simulink library "slident"  (Simulink 7.5)
settings: Solver=ode45  SolverMode=SingleTasking  StartTime=0.0  StopTime=10.0  RelTol=1e-3
values from neighbouring files (symbols this model uses):
  A = (pinv(R2(1:n,1:n)) * R2(1:n,n+1)).'    [ar.m]    (also in motor.m = s(1:2,1:2); n4sid.m = stab(A))
  B = s(1:2,3)    [motor.m]    (also in n4sid.m = B1)
  C = eye(2)    [motor.m]    (also in n4sid.m = conj(Un(1:ny,1:n)))
  D = D .* abs(ec{kexp}*ones(1,size(D,2)))    [arx.m]    (also in ivx.m = (OM(inda,:).').*(-Y*ones(1,na)); motor.m = [0;0]; n4sid.m = D1)
  data = pvset(data,'Name',Name)    [ar.m]    (also in arx.m = complex(data); arx_f.m = data(:,:,[]); etfe.m = iddata(data,[],T); idfilt.m = zfc{1})
  ts = ts{1}    [arx.m]    (also in arx_f.m = ts{1};[num1,den1]=tfdata(m0); arxstruc.m = pvget(z,'Ts'); iv4.m; n4sid.m)
  Ts = pvget(m0,'Ts')    [arx.m]    (also in arx_f.m = Ts{1}; idfilt.m = {1}; idresamp.m = pvget(data,'Ts'); iv4.m = Ts{1})
  X0 = [0;0]    [motor.m]    (also in n4sid.m = x(nxr,:).')
undefined symbols (not defined in the file or in its folder): Demos, gcbh, iddata, idss, idutils, offset, ph, slident2, Tdi, tsn
libraries: simulink x1
settings Model: RequirementInfo=9  Creator=greg  LastModifiedBy=rsingh  ExtModeAutoUpdateStatusClock=off
settings Model: ForwardingTableString=|
  | ||__slOldName__||slident/Output-error
  | model estimator.||__slNewName__||slident/Output-error
  | model estimator||__slOldName__||slident/Idnlgrey Model||__slNewName__||slident/Nonlinear Grey-Box Model

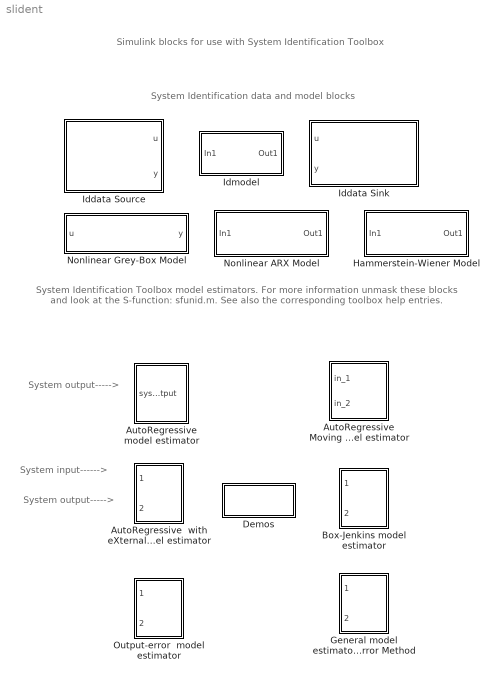
== system slident ==
  note: System Identification data and model blocks
  note: System output----->
  note: System input------>
  note: System output----->
  note: System Identification Toolbox model estimators. For more information
      | unmask these blocks and look at the  S-function: sfunid.m.
      | See also the corresponding toolbox help entries.
  note: Simulink blocks for use with
      | System Identification Toolbox
  AutoRegressive model estimator : Subsystem  AncestorBlock=slident2/AutoRegressive model estimator  mask(AR){order=3, HowOften=25, tso=0.05, npts=200, mn=, cbsim=1 step prediction}
      mask prompts: order "Orders of model [na]:"; HowOften "How often to update model (samples):"; tso "Sample time:"; npts "Length of data window (samples):"; mn "Model name:"; cbsim "Prediction horizon:"
      mask help:
      | Autoregressive model estimator for a scalar valued signal.
      | Model Name: Enter workspace variable name for resulting models. Leave empty for printout to MATLAB Command Window.
      | Choose prediction-horizon for the plots.
      mask init:
      | method='ar';
      | [ts,offset,ph,mn]=slidentinit(tso,cbsim,mn);
      mask Help:
      | AR block facilitates estimation of auto-regressive models in Simulink(R). Type "help ar" for more information. <br>
      | 
      | <p>
      | Hook a data source block to the input of the AR block. The estimated models are based on the latest data in the Data window. (initially padded with zeros). The model is re-estimated at the chosen rate. </p>
      | <p>
      | If a Model Name M is entered, the variable M will contain the estimated models
      | in a cell array, so that M{k,1} is the time associated with the k:th model and
      | M{k,2} is the actual model in IDPOLY format. The models can be used in Simulink(R) for simulation using the Idmodel block. They can also be simulated, analyzed and transformed in MATLAB Command Window using commands available with System Identification Toolbox(TM). For example, bode(M{:;2}) and step(M{:,2}) will show the bode plots and step responses of all the models.
      | </p>
      | <p>
      | If the model name is left empty, the models will be displayed in MATLAB Command Window. The properties of the models will also be displayed, on-line, as the  predicted output of the current model compared with the measured (actual) data. Choose between various prediction horizons using the Prediction horizon popup menu of the AR block. </p>
      | 
      | <p>
      | Results are displayed as the one step ahead predicted output versus the true output in graphical form.</p>
      mask StyleString: edit,edit,edit,edit,edit,popup(1 step prediction|5 step prediction|10 step prediction)
      mask Display:
      | disp('AR')
      | port_label('input',1,'y')
  AutoRegressive  with eXternal input model estimator : Subsystem  AncestorBlock=|  mask(ARX){order=[2 2 1], HowOften=25, tso=0.05, npts=200, mn=, cbsim=Simulation}
      | slident2/AutoRegressive 
      | with eXternal input
      | model estimator
      mask prompts: order "Orders of model [na nb nk]:"; HowOften "How often update model (samples):"; tso "Sample time:"; npts "Length of data window (samples):"; mn "Model name:"; cbsim "Simulation/Prediction:"
      mask help:
      | ARX model estimator.
      | Hook input 1 to system input.
      | Hook input 2 to system output.
      | Model Name: Enter workspace variable name for resulting models. Leave empty for printout to MATLAB Command Window.
      | Choose if presented model plots should be for simulation or prediction.
      mask init:
      | method='arx';
      | [ts,offset,ph,mn]=slidentinit(tso,cbsim,mn);
      mask Help:
      | ARX block facilitates estimation of auto-regressive models with exogenous inputs in Simulink(R). Type "help arx" for more information. <br>
      | 
      | <p>
      | Hook a data source representing input to an actual system to the first port of this block. Hook a data source representing measured output of the system to second port of the block. The estimated models are based on the latest data in the Data window. (initially padded with zeros). The model is re-estimated at the chosen rate. </p>
      | 
      | <p>
      | If a Model Name M is entered, the variable M will contain the estimated models
      | in a cell array, so that M{k,1} is the time associated with the k:th model and
      | M{k,2} is the actual model in IDPOLY format. The models can be used in Simulink(R) for simulation using the Idmodel block. They can also be simulated, analyzed and transformed in MATLAB Command Window using commands available with System Identification Toolbox(TM). For example, bode(M{:;2}) and step(M{:,2}) will show the bode plots and step responses of all the models. </p>
      | 
      | <p>
      | If the model name is left empty, the models will be displayed in MATLAB Command Window.
      | The properties of the models will also be displayed, on-line, as the simulated/predicted
      | output of the current model, compared with the measured (actual) output. Choose between
      | simulated outputs and predicted outputs over various prediction horizons. </p>
      mask StyleString: edit,edit,edit,edit,edit,popup(Simulation|1 step prediction|5 step prediction|10 step prediction)
      mask Display:
      | disp('ARX')
      | port_label('input',1,'u')
      | port_label('input',2,'y')
  AutoRegressive Moving Average with eXternal input model estimator : Subsystem  AncestorBlock=|  mask(ARMAX){order=[2 2 2 1], HowOften=25, tso=0.05, npts=200, mn=, cbsim=Simulation}
      | slident2/AutoRegressive Moving
      | Average with eXternal
      | input model estimator
      mask prompts: order "Orders of model [na nb nc nk]:"; HowOften "How often to update model (samples):"; tso "Sample time:"; npts "Length of data window (samples):"; mn "Model name:"; cbsim "Simulation/Prediction:"
      mask help:
      | ARMAX model estimator.
      | Hook input 1 to system input.
      | Hook input 2 to system output.
      | Model Name: Enter workspace variable name for resulting models. Leave empty for printout to MATLAB Command Window.
      | Choose if presented model plots should be for simulation or prediction.
      mask init:
      | method='armax';
      | [ts,offset,ph,mn]=slidentinit(tso,cbsim,mn);
      mask Help:
      | ARMAX block facilitates estimation of auto-regressive, moving average models with inputs (ARMAX) in Simulink(R). Type "help armax" for more information. <br>
      | 
      | <p>
      | Hook a data source representing input to an actual system to the first port of this block. Hook a data source representing measured output of the system to second port of the block. The estimated models are based on the latest data in the Data window. (initially padded with zeros). The model is re-estimated at the chosen rate. </p>
      | 
      | <p>
      | If a Model Name M is entered, the variable M will contain the estimated models
      | in a cell array, so that M{k,1} is the time associated with the k:th model and
      | M{k,2} is the actual model in IDPOLY format. The models can be used in Simulink(R) for simulation using the Idmodel block. They can also be simulated, analyzed and transformed in MATLAB Command Window using commands available with System Identification Toolbox(TM). For example, bode(M{:;2}) and step(M{:,2}) will show the bode plots and step responses of all the models. </p>
      | 
      | <p>
      | If the model name is left empty, the models will be displayed in MATLAB Command Window.
      | The properties of the models will also be displayed, on-line, as the simulated/predicted
      | output of the current model, compared with the measured (actual) output. Choose between
      | simulated outputs and predicted outputs over various prediction horizons. </p>
      mask StyleString: edit,edit,edit,edit,edit,popup(Simulation|1 step prediction|5 step prediction|10 step prediction)
      mask Display:
      | disp('ARMAX')
      | port_label('input',1,'u')
      | port_label('input',2,'y')
  Box-Jenkins model estimator : Subsystem  AncestorBlock=slident2/Box-Jenkins model estimator  mask(BJ){order=[2 2 2 2 1], HowOften=25, tso=0.05, npts=200, mn=, cbsim=Simulation}
      mask prompts: order "Orders of model [nb nc nd nf nk]:"; HowOften "How often to update model (samples):"; tso "Sample time:"; npts "Length of data window:"; mn "Model name:"; cbsim "Simulation/Prediction:"
      mask help:
      | Box-Jenkins model estimator.
      | Hook input 1 to system input.
      | Hook input 2 to system output.
      | Model Name: Enter workspace variable name for resulting models. Leave empty for printout to MATLAB Command Window.
      | Choose if presented model plots should be for simulation or prediction.
      mask init:
      | method='bj';
      | [ts,offset,ph,mn]=slidentinit(tso,cbsim,mn);
      mask Help:
      | BJ block facilitates estimation of Box-Jenkins models in Simulink(R). Type "help bj" for more information. <br>
      | 
      | <p>
      | Hook a data source representing input to an actual system to the first port of this block. Hook a data source representing measured output of the system to second port of the block. The estimated models are based on the latest data in the Data window. (initially padded with zeros). The model is re-estimated at the chosen rate. </p>
      | 
      | <p>
      | If a Model Name M is entered, the variable M will contain the estimated models
      | in a cell array, so that M{k,1} is the time associated with the k:th model and
      | M{k,2} is the actual model in IDPOLY format. The models can be used in Simulink(R) for simulation using the Idmodel block. They can also be simulated, analyzed and transformed in MATLAB Command Window using commands available with System Identification Toolbox(TM). For example, bode(M{:;2}) and step(M{:,2}) will show the bode plots and step responses of all the models. </p>
      | 
      | <p>
      | If the model name is left empty, the models will be displayed in MATLAB Command Window.
      | The properties of the models will also be displayed, on-line, as the simulated/predicted
      | output of the current model, compared with the measured (actual) output. Choose between
      | simulated outputs and predicted outputs over various prediction horizons. </p>
      mask StyleString: edit,edit,edit,edit,edit,popup(Simulation|1 step prediction|5 step prediction|10 step prediction)
      mask Display:
      | disp('BJ')
      | port_label('input',1,'u')
      | port_label('input',2,'y')
  Demos : Subsystem  AncestorBlock=slident2/Demos
      settings: OpenFcn=demo('toolbox','system identification')
      mask Display: disp('Demos')
  General model estimator using Predictive Error Method : Subsystem  AncestorBlock=|  mask(PEM){order=[2 2 2 2 2 1], HowOften=25, tso=0.05, npts=200, mn=, cbsim=Simulation}
      | slident2/General model
      | estimator using
      | Predictive Error Method
      mask prompts: order "Orders of model [na nb nc nd nf nk]:"; HowOften "How often to update model (samples):"; tso "Sample time:"; npts "Length of data window (samples):"; mn "Model name:"; cbsim "Simulation/Prediction:"
      mask help:
      | General SISO polynomial model estimator.
      | Hook input 1 to system input.
      | Hook input 2 to system output.
      | Model Name: Enter workspace variable name for resulting models. Leave empty for printout to MATLAB Command Window.
      | Choose if presented model plots should be for simulation or prediction.
      mask init:
      | method='pem';
      | [ts,offset,ph,mn]=slidentinit(tso,cbsim,mn);
      mask Help:
      | PEM block facilitates estimation of generic linear polynomial models in Simulink(R). Only linear, SISO models are supported. A generic polynomial structure has all its coefficients active so that the model equation is: A y(t) = B/F u(t-Nk) + C/D e(t). Type "help pem" and "help idpoly" for more information. <br>
      | <p>
      | Hook a data source representing input to an actual system to the first port of this block. Hook a data source representing measured output of the system to second port of the block. The estimated models are based on the latest data in the Data window. (initially padded with zeros). The model is re-estimated at the chosen rate. </p>
      | 
      | <p>
      | If a Model Name M is entered, the variable M will contain the estimated models
      | in a cell array, so that M{k,1} is the time associated with the k:th model and
      | M{k,2} is the actual model in IDPOLY format. The models can be used in Simulink(R) for simulation using the Idmodel block. They can also be simulated, analyzed and transformed in MATLAB Command Window using commands available with System Identification Toolbox(TM). For example, bode(M{:;2}) and step(M{:,2}) will show the bode plots and step responses of all the models. </p>
      | 
      | <p>
      | If the model name is left empty, the models will be displayed in MATLAB Command Window.
      | The properties of the models will also be displayed, on-line, as the simulated/predicted
      | output of the current model, compared with the measured (actual) output. Choose between
      | simulated outputs and predicted outputs over various prediction horizons. </p>
      mask StyleString: edit,edit,edit,edit,edit,popup(Simulation|1 step prediction|5 step prediction|10 step prediction)
      mask Display:
      | disp('PEM')
      | port_label('input',1,'u')
      | port_label('input',2,'y')
  Hammerstein-Wiener Model : Subsystem  mask(Hammerstein-Wiener Model){sys=, IC=Zero, X0i=0}
      mask prompts: sys "Model"; IC "Initial conditions:"; X0i "Specify a vector of state values"
      mask help:
      | Simulate a Hammerstein-Wiener (idnlhw) model. Enter a valid variable or expression representing an idnlhw model for the field "Model". The initial conditions for simulation can be specified using one of the following ways:
      | 1. Use "Zero" to use a value of zero for all initial state values.
      | 2. Specify the initial state values explicitly as a numerical vector for the linear block of the idnlhw model. Click on Help button for information on computation of initial states.
      mask init:
      | MaskVal = get_param(gcb,'MaskValues');
      | sysname = MaskVal{1};
      | if isa(sys,'idnlhw')
      |     %sysname = MaskVal{1};
      | else
      |     if isempty(sysname)
      |         sysname = 'IDNLHW MODEL';
      |     else
      |         sysname = '???';
      |     end
      |     sys = [];
      |     X0i = [];
      | end
      | if any(strcmp(get_param(bdroot(gcb),'SimulationStatus'),{'initializing','updating'}))
      |     lwarn = lastwarn;warn = warning('off');
      |     try
      |         [A,B,C,D,X0,Ts,WarnMsg] = idnlhwmaskinit('initialization',gcb,sys,IC,X0i);
      |         warning(warn);lastwarn(lwarn);
      |         warning(WarnMsg)
      |     catch E
      |         sys = [];
      |         X0i = [];
      |         sysname = '???';
      |         A = []; B = []; C = []; D = []; X0 = []; Ts = 1;
      |         warning(warn);lastwarn(lwarn);
      |         throw(E)
      |     end
      | end
      mask Help:
      | <p>Hammerstein-Wiener block simulates a nonlinear Hammerstein-Wiener (idnlhw) model. Type "help idnlhw" or "help nlhw" to see how to create a Hammerstein-Wiener model.  For more information, refer to the documentation on Hammerstein-Wiener models of System Identification Toolbox(TM). </p>
      | 
      | Specify the name of an idnlhw model for "Model". Simulation of the idnlhw model also requires specification of initial conditions. Initial conditions for this model are same as the initial states of the linear block that is embedded in the structure of the idnlhw model. Initial conditions may be specified in two ways:
      | <li> Zero value (default): Use this option to use a value of zero for all of the model's initial states.</li>
      | <li> Initial state values: Enter a vector of length equal to the number of states of the linear block in the corresponding edit field.</li>
      | <br>
      | The property "LinearModel" of the idnlhw object stores the linear block of the model as an IDPOLY or IDSS object. The states of the Hammerstein-Wiener model correspond to those of
      | this linear block. You may use "findop" and "findstates" commands to compute the states from specifications such as known past I/O values, steady-state conditions or values at a certain time from a previous simulation.
      | Type "help idnlhw/findop" or "help idnlhw/findstates" for more information.
      mask StyleString: edit,popup(Zero|State values),edit
      mask CallbackString:
      | idnlhwmaskinit('maskparamcallback',gcb)|maskStr = get_param(gcb,'MaskValues');
      | if strcmp(maskStr{2}(1),'S')
      |     % Set the visibility of all parameters on when
      |     % option "State values" is selected in the pop-up.
      |     set_param(gcb,'MaskVisibilities',{'on';'on';'on'});
      | else
      |     % Turn off the visibility of the X0i field
      |     % when option "State values" is not selected.
      |     set_param(gcb,'MaskVisibilities',{'on';'on';'off'});
      | end|
      mask Display: disp(sysname)
  Iddata Sink : Subsystem  InitFcn=idutils.iddataSinkManager('register', gcbh, get_param(gcb,'datasetname'))  StartFcn=idutils.iddataSinkStartFcnCallback(gcs)  mask(IDDATA Sink){datasetname=data, Ts=0.1, isu=off, isy=off}
      mask prompts: datasetname "IDDATA Name"; Ts "Sample Time (sec.)"; isu "InputPresent"; isy "OutputPresent"
      mask help: Enter in a name of a variable for which you would like the IDDATA data object be saved. The sample time is the rate that the data will be sampled.
      mask init:
      | [isu isy] = iddsink(gcb);
      mask Help:
      | Enter in a name of a variable for which you would like the IDDATA data object be saved.
      | 
      | The sample time is the rate that the data will be sampled.
      mask Display:
      | disp('IDDATA SINK')
      | port_label('input',1,'Input')
      | port_label('input',2,'Output')
  Iddata Source : Subsystem  mask(Iddata InputOutput){iddataobj=iddata(1,1)}
      mask prompts: iddataobj "IDDATA object"
      mask help:
      | This block allows to import IDDATA object from the MATLAB Workspace.
      |
      | The first output port of the block corresponds to the input signal of the IDDATA object and the second output port corresponds to the output signal.
      |
      | Enter an IDDATA object in the edit field.
      mask init:
      | warn = warning('off'); 
      | try
      |     [Ts,TimeUnit,dataname] = iddsrc(gcb,iddataobj);
      | catch E
      |     iddataobj = [];
      |     dataname = '???';
      |     warning(warn); 
      |     throw(E)
      | end
      | warning(warn)
      mask Help:
      | This block allows to import IDDATA object from the MATLAB Workspace.
      | <p>
      | The output ports of the block correspond  to the input and output signals of the IDDATA object.
      | <p>
      | Enter an IDDATA object in the edit field of the dialog.
      | <p>
      | The IDDATA block will automatically adjust to objects with input or output only.
      | <p>
      | The IDDATA object must contain just one experiment. Enter getexp(data,kexp) for a multi-experiment
      | object to select experiment number kexp. The intersample behavior of the input datais ignored and is always
      | assumed to be "first order hold" when used n the Iddata Source block.
      | <p>
      | Note that by default the start time ("Tstart") of an IDDATA object is not zero; it is equal to "Ts",
      | the sampling interval of the data. However, a Simulink model's default simulation start time is zero. For times
      | less than the value of Tstart, the Iddata Source block will supply a value of zero for signal values. In order to
      | have the Iddata Source block supply data samples right from the start of the simulation, it is recommended to
      | set the value of the "Tstart" property of the data object to be same at the start time in Simulink model.
      | For default settings, this implies setting Tstart to zero.
      mask Display:
      | disp(dataname)
      | port_label('output',1,'Input')
      | port_label('output',2,'Output')
  "Idmodel " : Subsystem  mask(Idmodel Block){sys=idss(-1,1,1,0), IC=0, noi=on, seed=}
      mask prompts: sys "idmodel variable"; IC "Initial state (state space only: 'z', 'm', or vector )"; noi "Add noise"; seed "Noise seed(s).  Default empty"
      mask help:
      | Enter any Idmodel object (Idpoly, Idss, Idarx, Idgrey or Idproc).
      | For simulations  with noise, Seed(s) may be left empty for random restarts.
      | Enter as many seeds as there are outputs for specific realizations.
      mask init:
      | warn = warning('off'); [lw,lwid] = lastwarn;
      | try
      |     [A,B,C,D,Ts,Tdi,X0,tsn,variance,ActSeed,sysname,noi1]=idmdlmask('InitializeData',gcb,sys,IC,noi,seed);
      |     idmdlmask('UpdateDiagram',gcb,Ts,noi1);
      | catch E
      |     sys = [];
      |     IC = [];
      |     sysname = '???';
      |     warning(warn); lastwarn(lw,lwid);
      |     throw(E)
      | end
      | warning(warn); lastwarn(lw,lwid);
      mask Help:
      | The IDMODEL  block 	accepts any IDMODEL defined in the System Identification Toolbox: IDPOLY, IDSS,
      | IDGREY, IDARX and IDPROC. <p><P>
      | 
      | In the editiable text box enter the name of any IDMODEL in workspace.<p><p>
      | 
      |  For IDMODELS in state-space (IDSS and IDGREY) the initial state vector may be
      | specified. Use 'z' (within quotes) or 0 for zero initial conditions, use 'm' for the
      | Model's own initial state (I.e. MOD.X0) or specify the initial state  as a vector.<p><p>
      | 
      | To add noise to the simulation, check the corresponding box. Noise will be
      | added in accordance with the models noise specifications, i.e. MOD.NoiseVariance and
      | the matrices or polynomials that determine the color of the additive noise. <p><p>
      | 
      | For continuous time models the variance of the momentary noise term is infinite
      | in theory. You will see an appropriately bandlimited version, taking into account
      | the natural time constants of the system. You may think of the resulting simulated output
      | being filtered with a low-pass filter with a pass-band that does not distort the dynamics
      | from the input.<p><p>
      | 
      | IDMODELS with time-delays (MOD.InputDelay nonzero) are properly treated. Discrete time
      | models are convereted into models which take care of the delay explicitly, (thereby
      | extending also X0). For continuous time models a transport delay block is used.
      mask CallbackString: idmdlmask('MaskLTICallback',gcb)||idmdlmask('MaskLTICallback',gcb)|
      mask Display: disp(sysname)
  Nonlinear ARX Model : Subsystem  mask(Nonlinear ARX Model){sys=, ICspec=Input and output values, X0=0, U0=0, Y0=0}
      mask prompts: sys "Model"; ICspec "Initial conditions:"; X0 "Vector of state values:"; U0 "Input level:"; Y0 "Output level:"
      mask help:
      | Simulate a nonlinear ARX (idnlarx) model. Enter a valid variable or expression representing an idnlarx model for the field "Model". The initial conditions for simulation can be specified in one of the following ways:
      | 1. Specify steady-state (equilibrium) input and output signal levels.
      | 2. Specify an initial state vector. Click on Help button for information on computation of initial states.
      mask init:
      | MaskVal = get_param(gcb,'MaskValues');
      | sysname = MaskVal{1};
      | if isa(sys,'idnlarx')
      |     maskEn = get_param(gcb,'MaskEnables');
      |     nu = size(sys,'nu');
      |     fInp = find_system(gcb,'FollowLinks','on','LookUnderMasks','all',...
      |         'SearchDepth',1,'Name','In1');
      | 
      |     if nu>0 && isempty(fInp)
      |         add_block('built-in/Inport',[gcb,'/In1'],'Position',[20   133    50   147])
      |     elseif nu==0 && ~isempty(fInp)
      |         delete_block(fInp);
      |     end
      |     %{
      |     if nu==0
      |         maskEn{4} = 'off';
      |     else
      |         maskEn{4} = 'on';
      |     end
      |     %}
      | 
      |     set_param(gcb,'MaskEnables',maskEn);
      | 
      | else
      |     if isempty(sysname)
      |         sysname = 'IDNLARX MODEL';
      |     else
      |         sysname = '???';
      |     end
      |     sys = [];
      |     U0 = [];
      |     Y0 = [];
      |     X0 = [];
      |     Nx = 0;
      |     
      | end
      | 
      | if any(strcmp(get_param(bdroot(gcb),'SimulationStatus'),{'initializing','updating'}))
      |     lwarn = lastwarn;warn = warning('off');
      |     try
      |         [X0,Ts,WarnMsg] = idnlarxmaskinit('initialization',gcb,sys,ICspec,X0,U0,Y0);
      |         Nx = length(X0);
      |         warning(warn);lastwarn(lwarn);
      |         for i = 1:size(WarnMsg,1)
      |             warning(WarnMsg{i,1},WarnMsg{i,2})
      |         end
      |     catch E
      |         sys = [];
      |         U0 = [];
      |         Y0 = [];
      |         sysname = '???';
      |         X0 = [];
      |         Nx = 0;
      |         warning(warn);lastwarn(lwarn);
      |         throw(E)
      |     end
      | end
      mask Help:
      | <p>Nonlinear ARX block simulates a nonlinear ARX (idnlarx) model. Type "help idnlarx" or "help nlarx" to see how to create a nonlinear ARX model.  For more information, refer to the documentation on Nonlinear ARX models of System Identification Toolbox(TM). </p>
      | 
      | Specify the name of an idnlarx model for "Model". Simulation of the idnlarx model also requires specification of initial conditions.
      | The initial conditions may be specified in two ways:
      | <li> As input and output values: If the model is assumed or known to be in a state of equilibrium before the start of simulation,
      | you may specify the constant equilibrium values for all the model's input and output channels.
      | Enter a vector of length equal to the number of model's inputs for the field "Input level".
      | Similarly, enter a vector of length equal to the number of model's outputs for the field "Output level".
      | If a scalar is entered in either fields, that scalar is taken as the signal value for all the channels in that field.</li>
      | <li> As initial state values: The states of the model are defined as delayed samples of model's I/O variables.
      | The number of states is determined by the sum total of maximum delays in all I/O channels.
      | You may use commands such as "data2state", "findop" and "findstates" to compute the initial state values from specifications
      | such as known past I/O values, steady-state conditions or values at a certain time from a previous simulation.
      | Type "help data2state", "help idnlarx/findop" or "help idnlarx/findstates" for more information.</li>
      mask StyleString: edit,popup(Input and output values|State values),edit,edit,edit
      mask CallbackString:
      | idnlarxmaskinit('maskparamcallback',gcb)
      | |maskStr = get_param(gcb,'MaskValues');
      | if strcmp(maskStr{2}(1),'S')
      |     % "State values" option
      |     set_param(gcb,  'MaskVisibilities',   {'on';'on';'on';'off';'off'});
      |     %set_param(gcb,  'MaskEnables',        {'on';'on';'on';'off';'off'});
      | elseif strcmp(maskStr{2}(1),'I')
      |     % "Input and output values" option (default)
      |     set_param(gcb,  'MaskVisibilities',   {'on';'on';'off';'on';'on'});
      |     %set_param(gcb,  'MaskEnables',        {'on';'on';'off';'on';'on'});
      | end|||
      mask Display: disp(sysname)
  Nonlinear Grey-Box Model : Subsystem  mask(Nonlinear Grey-Box Model){nlsys=, X0='m'}
      mask prompts: nlsys "IDNLGREY model"; X0 "Initial state ('z', 'm', vector or structure  array); default is 'm'"
      mask help: Enter name of an IDNLGREY object and, optionally, an initial state X0.
      mask init:
      | MaskVal = get_param(gcb,'MaskValues');
      | sysname = MaskVal{1};
      | if isempty(sysname)
      |     sysname = 'IDNLGREY MODEL';
      | elseif ~isa(nlsys,'idnlgrey')
      |     sysname = '???';
      | end
      mask Help:
      | The IDNLGREY  block accepts any IDNLGREY model as defined in the System Identification Toolbox.<p><P>
      | 
      | In the editiable text box enter the name of any IDNLGREY model in workspace.<p><p>
      | 
      | The initial state vector may be specified. Use
      |    <li>'zero' (or just 'z' within quotes) for zero initial conditions.
      |   <li> 'model' (or just 'm') for the model's own internal initial state.
      |    <li> a vector of proper size.
      |    <li>an initial state structure array with fields 'Name', 'Unit', 'Value', 'Minimum', 'Maximum' and 'isFixed'; see help on @idnlgrey/sim for more details on how to create this structure.
      mask Display: disp(sysname)
  Output-error  model estimator : Subsystem  AncestorBlock="slident2/Output-error  model estimator."  mask(OE){order=[2 2 1], HowOften=25, tso=0.05, npts=200, mn=, cbsim=Simulation}
      mask prompts: order "Orders of model [nb nf nk]:"; HowOften "How often to update model (samples):"; tso "Sample time:"; npts "Length of data window (samples):"; mn "Model name:"; cbsim "Simulation/Prediction:"
      mask help:
      | Output-error model estimator.
      | Hook input 1 to system input.
      | Hook input 2 to system output.
      | Model Name: Enter workspace variable name for resulting models. Leave empty for printout to MATLAB Command Window.
      | Choose if presented model plots should be for simulation or prediction.
      mask init:
      | method='oe';
      | [ts,offset,ph,mn]=slidentinit(tso,cbsim,mn);
      mask Help:
      | BJ block facilitates estimation of Output-Error models in Simulink(R). Type "help oe" for more information. <br>
      | 
      | <p>
      | Hook a data source representing input to an actual system to the first port of this block. Hook a data source representing measured output of the system to second port of the block. The estimated models are based on the latest data in the Data window. (initially padded with zeros). The model is re-estimated at the chosen rate. </p>
      | 
      | <p>
      | If a Model Name M is entered, the variable M will contain the estimated models
      | in a cell array, so that M{k,1} is the time associated with the k:th model and
      | M{k,2} is the actual model in IDPOLY format. The models can be used in Simulink(R) for simulation using the Idmodel block. They can also be simulated, analyzed and transformed in MATLAB Command Window using commands available with System Identification Toolbox(TM). For example, bode(M{:;2}) and step(M{:,2}) will show the bode plots and step responses of all the models. </p>
      | 
      | <p>
      | If the model name is left empty, the models will be displayed in MATLAB Command Window.
      | The properties of the models will also be displayed, on-line, as the simulated/predicted
      | output of the current model, compared with the measured (actual) output. Choose between
      | simulated outputs and predicted outputs over various prediction horizons. </p>
      mask StyleString: edit,edit,edit,edit,edit,popup(Simulation|1 step prediction|5 step prediction|10 step prediction)
      mask Display:
      | disp('OE')
      | port_label('input',1,'u')
      | port_label('input',2,'y')

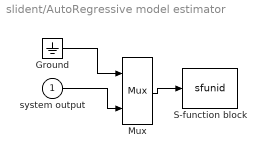
== system slident/AutoRegressive model estimator ==
  system output : Inport  OutDataType=sfix(16)  OutScaling=2^0
  Ground : Ground
  Mux : Mux  Inputs=2
  S-function block : S-Function  FunctionName=sfunid  Parameters=order,npts,HowOften,offset,ts,method,mn,ph  EnableBusSupport=off
      settings: DeleteFcn=sfunid([],[],[],'DeleteBlock')
  wires:
  Ground/1 -> Mux/1
  system output/1 -> Mux/2
  Mux/1 -> S-function block/1

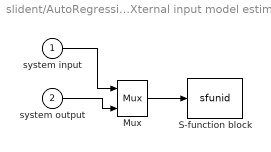
== system slident/AutoRegressive  with eXternal input model estimator ==
  system input : Inport  OutDataType=sfix(16)  OutScaling=2^0
  system output : Inport  Port=2  OutDataType=sfix(16)  OutScaling=2^0
  Mux : Mux  Inputs=2
  S-function block : S-Function  FunctionName=sfunid  Parameters=order,npts,HowOften,offset,ts,method,mn,ph  EnableBusSupport=off
      settings: DeleteFcn=sfunid([],[],[],'DeleteBlock')
  wires:
  system input/1 -> Mux/1
  system output/1 -> Mux/2
  Mux/1 -> S-function block/1

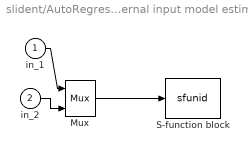
== system slident/AutoRegressive Moving Average with eXternal input model estimator ==
  in_1 : Inport  OutDataType=sfix(16)  OutScaling=2^0
  in_2 : Inport  Port=2  OutDataType=sfix(16)  OutScaling=2^0
  Mux : Mux  Inputs=2
  S-function block : S-Function  FunctionName=sfunid  Parameters=order,npts,HowOften,offset,ts,method,mn,ph  EnableBusSupport=off
      settings: DeleteFcn=sfunid([],[],[],'DeleteBlock')
  wires:
  Mux/1 -> S-function block/1
  in_1/1 -> Mux/1
  in_2/1 -> Mux/2

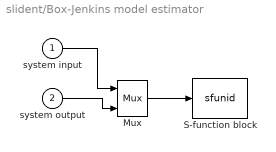
== system slident/Box-Jenkins model estimator ==
  system input : Inport  OutDataType=sfix(16)  OutScaling=2^0
  system output : Inport  Port=2  OutDataType=sfix(16)  OutScaling=2^0
  Mux : Mux  Inputs=2
  S-function block : S-Function  FunctionName=sfunid  Parameters=order,npts,HowOften,offset,ts,method,mn,ph  EnableBusSupport=off
      settings: DeleteFcn=sfunid([],[],[],'DeleteBlock')
  wires:
  Mux/1 -> S-function block/1
  system output/1 -> Mux/2
  system input/1 -> Mux/1

== system slident/Demos ==

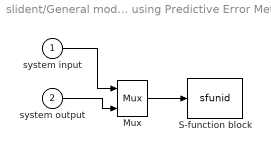
== system slident/General model estimator using Predictive Error Method ==
  system input : Inport  OutDataType=sfix(16)  OutScaling=2^0
  system output : Inport  Port=2  OutDataType=sfix(16)  OutScaling=2^0
  Mux : Mux  Inputs=2
  S-function block : S-Function  FunctionName=sfunid  Parameters=order,npts,HowOften,offset,ts,method,mn,ph  EnableBusSupport=off
      settings: DeleteFcn=sfunid([],[],[],'DeleteBlock')
  wires:
  Mux/1 -> S-function block/1
  system output/1 -> Mux/2
  system input/1 -> Mux/1

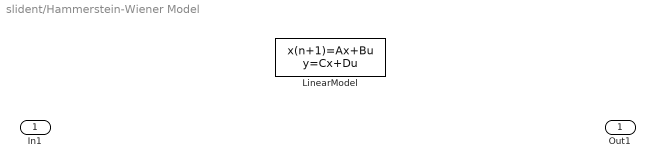
== system slident/Hammerstein-Wiener Model ==
  In1 : Inport  OutDataType=sfix(16)  OutScaling=2^0
  LinearModel : DiscreteStateSpace  A=A  B=B  C=C  D=D  X0=X0  SampleTime=Ts
  Out1 : Outport  OutDataType=sfix(16)  OutScaling=2^0

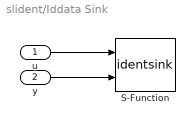
== system slident/Iddata Sink ==
  u : Inport  OutDataType=sfix(16)  OutScaling=2^0
  y : Inport  Port=2  OutDataType=sfix(16)  OutScaling=2^0
  S-Function : S-Function  FunctionName=identsink  Parameters=datasetname Ts isu isy  EnableBusSupport=off
  wires:
  y/1 -> S-Function/2
  u/1 -> S-Function/1

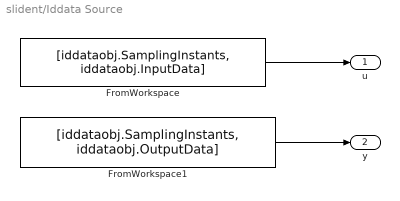
== system slident/Iddata Source ==
  FromWorkspace : FromWorkspace  VariableName=[iddataobj.SamplingInstants, iddataobj.InputData]  SampleTime=iddataobj.Ts  OutputAfterFinalValue=Setting to zero
  FromWorkspace1 : FromWorkspace  VariableName=[iddataobj.SamplingInstants, iddataobj.OutputData]  SampleTime=iddataobj.Ts  OutputAfterFinalValue=Setting to zero
  u : Outport  OutDataType=sfix(16)  OutScaling=2^0
  y : Outport  Port=2  OutDataType=sfix(16)  OutScaling=2^0
  wires:
  FromWorkspace1/1 -> y/1
  FromWorkspace/1 -> u/1

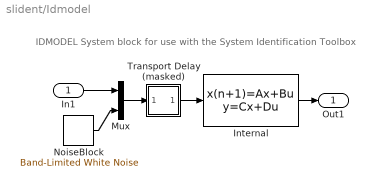
== system slident/Idmodel  ==
  note: IDMODEL System block
      | for use with the
      | System Identification Toolbox
  In1 : Inport  OutDataType=sfix(16)  OutScaling=2^0
  Internal : DiscreteStateSpace  A=A  B=B  C=C  D=D  X0=X0  SampleTime=Ts
  Mux : Mux  Inputs=2
  NoiseBlock : simulink/Sources/Band-Limited White Noise  Tag=NoiseBlock  SystemSampleTime=-1  Cov=variance  Ts=tsn  seed=ActSeed
  Transport Delay (masked) : Subsystem  Tag=InputDelayBlock  AncestorBlock=|  mask(Transport Delay (masked)){Td=Tdi, u0=0, bufsize=1024}
      | identextras/Transport Delay
      | (masked)
      mask prompts: Td "Delay Time"; u0 "Initial Input"; bufsize "Initial Buffer Size"
      mask help: Transport Delay, with direct feedthrough when Delay Time is equal to zero.
      mask init:
      | df = get_param(bdroot,'dirty');
      | iddfthru(gcb, Td, u0, bufsize);
      | set_param(bdroot,'dirty',df)
      mask Help: See Transport Delay for more information.
      mask Display: plot([0 1],[0.5 0.5])
  Out1 : Outport  OutDataType=sfix(16)  OutScaling=2^0
  wires:
  Transport Delay (masked)/1(Outport) -> Internal/1
  Mux/1 -> Transport Delay (masked)/1(Inport)
  Internal/1 -> Out1/1
  In1/1 -> Mux/1
  NoiseBlock/1 -> Mux/2

== system slident/Nonlinear ARX Model ==
  In1 : Inport  OutDataType=sfix(16)  OutScaling=2^0
  Out1 : Outport  OutDataType=sfix(16)  OutScaling=2^0

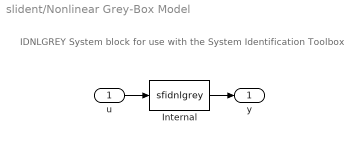
== system slident/Nonlinear Grey-Box Model ==
  note: IDNLGREY System block
      | for use with the
      | System Identification Toolbox
  u : Inport  OutDataType=sfix(16)  OutScaling=2^0
  Internal : S-Function  FunctionName=sfidnlgrey  Parameters=nlsys, X0  EnableBusSupport=off
  y : Outport  OutDataType=sfix(16)  OutScaling=2^0
  wires:
  Internal/1 -> y/1
  u/1 -> Internal/1

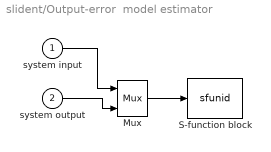
== system slident/Output-error  model estimator ==
  system input : Inport  OutDataType=sfix(16)  OutScaling=2^0
  system output : Inport  Port=2  OutDataType=sfix(16)  OutScaling=2^0
  Mux : Mux  Inputs=2
  S-function block : S-Function  FunctionName=sfunid  Parameters=order,npts,HowOften,offset,ts,method,mn,ph  EnableBusSupport=off
      settings: DeleteFcn=sfunid([],[],[],'DeleteBlock')
  wires:
  system input/1 -> Mux/1
  system output/1 -> Mux/2
  Mux/1 -> S-function block/1

== system slident/Idmodel /Transport Delay (masked) ==
  Inport : Inport  OutDataType=sfix(16)  OutScaling=2^0
  Outport : Outport  OutDataType=sfix(16)  OutScaling=2^0
  wires:
  Inport/1 -> Outport/1
